simulink model "Yaw_Rate_Damper"  (R2024b)
settings: Solver=VariableStepAuto  StartTime=0.0  StopTime=40  RelTol=1e-3
undefined symbols (not defined in the file or in its folder): Kp_a
libraries: slpidlib x2
settings Model: Creator=GH-X-ST  LastModifiedBy=GH-X-ST

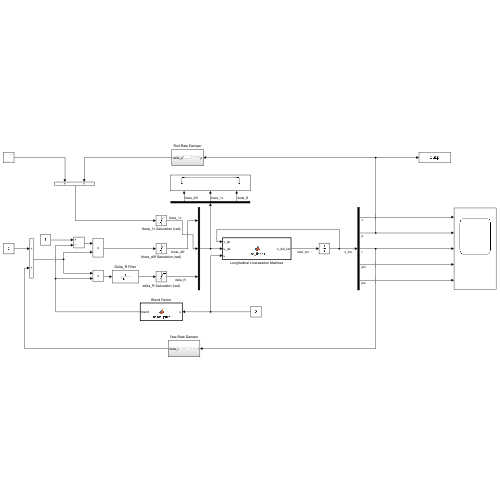
[thumbnail: Simulink's stored preview of the top-level diagram]
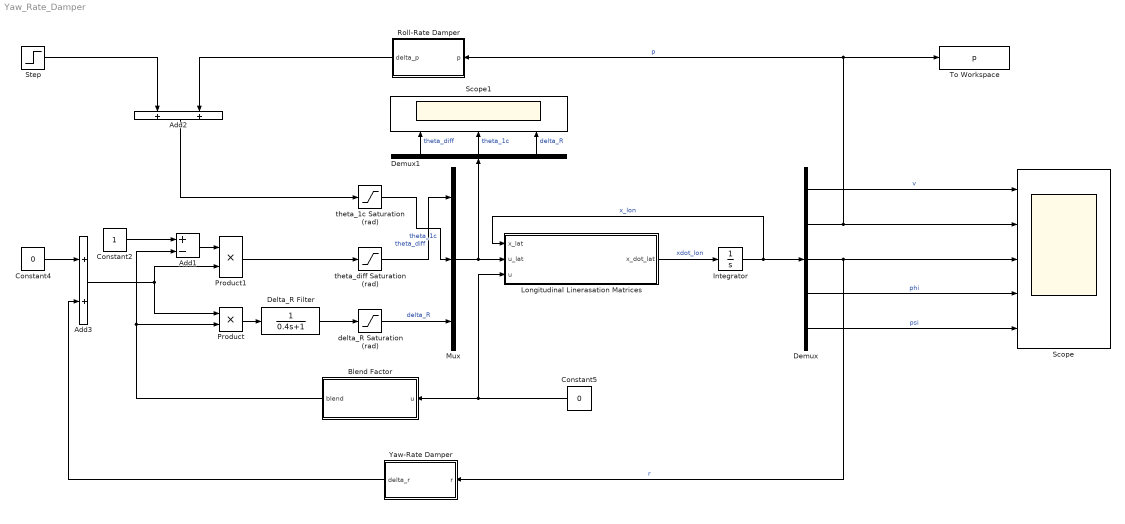
== system Yaw_Rate_Damper ==
  Add1 : Sum  Inputs=+-
  Add2 : Sum
  Add3 : Sum
  Blend Factor : MATLAB Function  TreatAsAtomicUnit=on
  Constant2 : Constant
  Constant4 : Constant  Value=0
  Constant5 : Constant  Value=0
  Delta_R Filter : TransferFcn  Denominator=[0.4 1]
  Demux : Demux  Outputs=5
  Demux1 : Demux  Outputs=3
  Integrator : Integrator  InitialCondition=[0;0;0;0;0]
  Longitudinal Linerasation Matrices : MATLAB Function  TreatAsAtomicUnit=on
  Mux : Mux  Inputs=3
  Product : Product
  Product1 : Product
  Roll-Rate Damper : Subsystem
  Scope : Scope  NumInputPorts=5
  Scope1 : Scope  NumInputPorts=3
  Step : Step  After=0.005  SampleTime=0
  To Workspace : ToWorkspace  VariableName=p  SaveFormat=Timeseries  SampleTime=-1
  Yaw-Rate Damper : Subsystem
  delta_R Saturation (rad) : Saturate  UpperLimit=deg2rad(11)  LowerLimit=deg2rad(-11)
  theta_1c Saturation (rad) : Saturate  UpperLimit=deg2rad(3)  LowerLimit=deg2rad(-3)
  theta_diff Saturation (rad) : Saturate  UpperLimit=deg2rad(5)  LowerLimit=deg2rad(-5)
  wires:
  Longitudinal Linerasation Matrices/1(x_dot_lat) -> Integrator/1  "xdot_lon"
  Integrator/1 -> Longitudinal Linerasation Matrices/1(x_lat), Demux/1  "x_lon"
  Demux/1 -> Scope/1  "v"
  Demux/2 -> Roll-Rate Damper/1(p), To Workspace/1, Scope/2  "p"
  Demux/3 -> Yaw-Rate Damper/1(r), Scope/3  "r"
  Demux/4 -> Scope/4  "phi"
  delta_R Saturation (rad)/1 -> Mux/3  "delta_R"
  Blend Factor/1(blend) -> Add1/2, Product/2
  Add3/1 -> Product1/2, Product/1
  Constant2/1 -> Add1/1
  Add1/1 -> Product1/1
  Mux/1 -> Demux1/1, Longitudinal Linerasation Matrices/2(u_lat)
  Demux1/3 -> Scope1/3  "delta_R"
  Demux1/2 -> Scope1/2  "theta_1c"
  Demux1/1 -> Scope1/1  "theta_diff"
  Product1/1 -> theta_diff Saturation (rad)/1
  Product/1 -> Delta_R Filter/1
  Delta_R Filter/1 -> delta_R Saturation (rad)/1
  Demux/5 -> Scope/5  "psi"
  Yaw-Rate Damper/1(delta_r) -> Add3/2
  Constant4/1 -> Add3/1
  theta_diff Saturation (rad)/1 -> Mux/1  "theta_diff"
  theta_1c Saturation (rad)/1 -> Mux/2  "theta_1c"
  Constant5/1 -> Longitudinal Linerasation Matrices/3(u), Blend Factor/1(u)
  Step/1 -> Add2/1
  Roll-Rate Damper/1(delta_p) -> Add2/2
  Add2/1 -> theta_1c Saturation (rad)/1

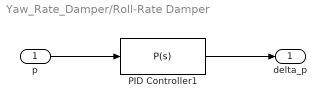
== system Yaw_Rate_Damper/Roll-Rate Damper ==
  p : Inport
  PID Controller1 : slpidlib/PID Controller  Controller=P  Form=Parallel  TimeDomain=Continuous-time  UseExternalTs=off  SampleTime=-1  IntegratorMethod=Forward Euler  FilterMethod=Forward Euler  ControllerParametersSource=internal  P=Kp_a  I=0.005  UseKiTs=off  D=0.005  UseExternalDerivativeSource=on  N=100  UseFilter=on  TunerSelectOption=Transfer Function Based (PID Tuner App)  InitialConditionSource=internal  InitialConditionForIntegrator=0  InitialConditionForFilter=0  DifferentiatorICPrevScaledInput=0  ExternalReset=none  TrackingMode=off  Kt=1  LimitOutput=on  SatLimitsSource=internal  UpperSaturationLimit=1  LowerSaturationLimit=-1  LinearizeAsGain=on  AntiWindupMode=none  Kb=1  LimitIntegrator=off  UpperIntegratorSaturationLimit=inf  LowerIntegratorSaturationLimit=-inf  POutMin=[]  POutMax=[]  IOutMin=[]  IOutMax=[]  DOutMin=[]  DOutMax=[]  NOutMin=[]  NOutMax=[]  SumOutMin=[]  SumOutMax=[]  SaturationOutMin=[]  SaturationOutMax=[]  PParamMin=[]  PParamMax=[]  IParamMin=[]  IParamMax=[]  DParamMin=[]  DParamMax=[]  NParamMin=[]  NParamMax=[]  KbParamMin=[]  KbParamMax=[]  KtParamMin=[]  KtParamMax=[]  KbOutMin=[]  KbOutMax=[]  KtOutMin=[]  KtOutMax=[]  IntegratorOutMin=[]  IntegratorOutMax=[]  FilterOutMin=[]  FilterOutMax=[]  SumI1OutMin=[]  SumI1OutMax=[]  SumI2OutMin=[]  SumI2OutMax=[]  SumI3OutMin=[]  SumI3OutMax=[]  SumI4OutMin=[]  SumI4OutMax=[]  SumDOutMin=[]  SumDOutMax=[]  DifferentiatorOutMin=[]  DifferentiatorOutMax=[]  FilterDiffOutCoefMin=[]  FilterDiffOutCoefMax=[]  ReciprocalOutMin=[]  ReciprocalOutMax=[]  SumDenOutMin=[]  SumDenOutMax=[]  SumNumOutMin=[]  SumNumOutMax=[]  DivideOutMin=[]  DivideOutMax=[]  UdiffTsProdOutMin=[]  UdiffTsProdOutMax=[]  NTsProdOutMin=[]  NTsProdOutMax=[]  UintegralTsProdOutMin=[]  UintegralTsProdOutMax=[]  UngainTsProdOutMin=[]  UngainTsProdOutMax=[]  ClampingZeroOutDataTypeStr=Inherit: Inherit via back propagation  ClampingZeroOutMin=[]  ClampingZeroOutMax=[]  FilterDenConstantOutDataTypeStr=Inherit: Inherit via back propagation  FilterDenConstantOutMin=[]  FilterDenConstantOutMax=[]  PCopyOutDataTypeStr=Inherit: Inherit via back propagation  PCopyOutMin=[]  PCopyOutMax=[]  NCopyOutDataTypeStr=Inherit: Inherit via back propagation  NCopyOutMin=[]  NCopyOutMax=[]  IntegratorContinuousStateAttributes=''  IntegratorStateMustResolveToSignalObject=off  IntegratorRTWStateStorageClass=Auto  FilterContinuousStateAttributes=''  FilterStateMustResolveToSignalObject=off  FilterRTWStateStorageClass=Auto  ParallelPVariant=InternalParameters  IdealPVariant=Disabled  IVariant=Disabled  DVariant=Disabled  IntegratorVariant=Disabled  SatVariant=Enabled  AWVariant=Disabled  PCopyVariant=Disabled  TRVariant=Disabled  FdbkBlocksVariant=Forward  IdealPFdbkVariant=Disabled  SatFdbkVariant=Disabled  DerivativeFilterVariant=Disabled  NVariant=Passthrough  NCopyVariant=Disabled_SignalSpec  FilterICVariant=Disabled  IntegratorICVariant=Disabled  ExternalResetVariant=Disabled  TRSumVariant=Passthrough  SumFdbkVariant=Disabled  SumVariant=Passthrough_P  TsampFilterVariant=InternalTs  TsampNgainVariant=Passthrough  TsampIntegralVariant=Disabled_SignalSpec  ExternalSaturationOutDataTypeStr=Inherit: Same as second input  DerivativeSourceVariant=Disabled  PreIntVariant=InternalPreInt
  delta_p : Outport
  wires:
  PID Controller1/1 -> delta_p/1
  p/1 -> PID Controller1/1

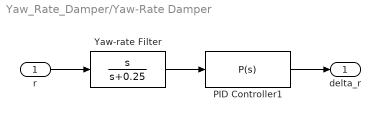
== system Yaw_Rate_Damper/Yaw-Rate Damper ==
  r : Inport
  PID Controller1 : slpidlib/PID Controller  Controller=P  Form=Parallel  TimeDomain=Continuous-time  UseExternalTs=off  SampleTime=-1  IntegratorMethod=Forward Euler  FilterMethod=Forward Euler  ControllerParametersSource=internal  P=0.01  I=0.005  UseKiTs=off  D=0.005  UseExternalDerivativeSource=on  N=100  UseFilter=on  TunerSelectOption=Transfer Function Based (PID Tuner App)  InitialConditionSource=internal  InitialConditionForIntegrator=0  InitialConditionForFilter=0  DifferentiatorICPrevScaledInput=0  ExternalReset=none  TrackingMode=off  Kt=1  LimitOutput=on  SatLimitsSource=internal  UpperSaturationLimit=1  LowerSaturationLimit=-1  LinearizeAsGain=on  AntiWindupMode=none  Kb=1  LimitIntegrator=off  UpperIntegratorSaturationLimit=inf  LowerIntegratorSaturationLimit=-inf  POutMin=[]  POutMax=[]  IOutMin=[]  IOutMax=[]  DOutMin=[]  DOutMax=[]  NOutMin=[]  NOutMax=[]  SumOutMin=[]  SumOutMax=[]  SaturationOutMin=[]  SaturationOutMax=[]  PParamMin=[]  PParamMax=[]  IParamMin=[]  IParamMax=[]  DParamMin=[]  DParamMax=[]  NParamMin=[]  NParamMax=[]  KbParamMin=[]  KbParamMax=[]  KtParamMin=[]  KtParamMax=[]  KbOutMin=[]  KbOutMax=[]  KtOutMin=[]  KtOutMax=[]  IntegratorOutMin=[]  IntegratorOutMax=[]  FilterOutMin=[]  FilterOutMax=[]  SumI1OutMin=[]  SumI1OutMax=[]  SumI2OutMin=[]  SumI2OutMax=[]  SumI3OutMin=[]  SumI3OutMax=[]  SumI4OutMin=[]  SumI4OutMax=[]  SumDOutMin=[]  SumDOutMax=[]  DifferentiatorOutMin=[]  DifferentiatorOutMax=[]  FilterDiffOutCoefMin=[]  FilterDiffOutCoefMax=[]  ReciprocalOutMin=[]  ReciprocalOutMax=[]  SumDenOutMin=[]  SumDenOutMax=[]  SumNumOutMin=[]  SumNumOutMax=[]  DivideOutMin=[]  DivideOutMax=[]  UdiffTsProdOutMin=[]  UdiffTsProdOutMax=[]  NTsProdOutMin=[]  NTsProdOutMax=[]  UintegralTsProdOutMin=[]  UintegralTsProdOutMax=[]  UngainTsProdOutMin=[]  UngainTsProdOutMax=[]  ClampingZeroOutDataTypeStr=Inherit: Inherit via back propagation  ClampingZeroOutMin=[]  ClampingZeroOutMax=[]  FilterDenConstantOutDataTypeStr=Inherit: Inherit via back propagation  FilterDenConstantOutMin=[]  FilterDenConstantOutMax=[]  PCopyOutDataTypeStr=Inherit: Inherit via back propagation  PCopyOutMin=[]  PCopyOutMax=[]  NCopyOutDataTypeStr=Inherit: Inherit via back propagation  NCopyOutMin=[]  NCopyOutMax=[]  IntegratorContinuousStateAttributes=''  IntegratorStateMustResolveToSignalObject=off  IntegratorRTWStateStorageClass=Auto  FilterContinuousStateAttributes=''  FilterStateMustResolveToSignalObject=off  FilterRTWStateStorageClass=Auto  ParallelPVariant=InternalParameters  IdealPVariant=Disabled  IVariant=Disabled  DVariant=Disabled  IntegratorVariant=Disabled  SatVariant=Enabled  AWVariant=Disabled  PCopyVariant=Disabled  TRVariant=Disabled  FdbkBlocksVariant=Forward  IdealPFdbkVariant=Disabled  SatFdbkVariant=Disabled  DerivativeFilterVariant=Disabled  NVariant=Passthrough  NCopyVariant=Disabled_SignalSpec  FilterICVariant=Disabled  IntegratorICVariant=Disabled  ExternalResetVariant=Disabled  TRSumVariant=Passthrough  SumFdbkVariant=Disabled  SumVariant=Passthrough_P  TsampFilterVariant=InternalTs  TsampNgainVariant=Passthrough  TsampIntegralVariant=Disabled_SignalSpec  ExternalSaturationOutDataTypeStr=Inherit: Same as second input  DerivativeSourceVariant=Disabled  PreIntVariant=InternalPreInt
  Yaw-rate Filter : TransferFcn  Numerator=[1 0]  Denominator=[1 0.25]
  delta_r : Outport
  wires:
  PID Controller1/1 -> delta_r/1
  Yaw-rate Filter/1 -> PID Controller1/1
  r/1 -> Yaw-rate Filter/1

== matlab function Yaw_Rate_Damper/Longitudinal Linerasation Matrices ==
  data: x_lat input; u_lat input; u input; x_dot_lat output
function x_dot_lat = Lat_linear(x_lat, u_lat, u)
% Author:
%   Hanchen Li (hl3422@ic.ac.uk)
%
% Inputs:
%   x_lat     - [v, p, r, phi, psi]
%   v         - Lateral velocity (m/s)
%   p         - Roll rate (rad/s)
%   r         - Yaw rate (rad/s)
%   phi       - Euler roll angle (rad)
%   psi       - Euler yaw angle (rad)
%
%   u_lat      - [theta_diff, theta_1c, delta_R]
%   theta_diff - Rotor collective difference (rad)
%   theta_1c   - Lateral cyclic (rad)
%   delta_R    - Rudder deflection (rad)
%
%   u         - Forward velocity (m/s)
%
% Outputs:
%   x_dot_lat

A_lat = ...
[-0.00723803596901745	0.766629187912504	0	9.80664998365558	0;
        -0.0220588605968897	2.33772683898305	0	0	0;
        -0.00849763594524569	0.895100650677353	0	0	0;
        0	1	-3.37129866355175e-20	0	0;
        0	0	1	0	0];

B_lat = ...
[3.23169927067643e-19	-5.17979000748556	0;
        39.4348460540525	-15.7950340421649	0;
        20.0367522163849	-6.04781748357008	0;
        0	0	0;
        0	0	0];

%% 3 Output
x_dot_lat = A_lat * x_lat + B_lat * u_lat;

end

== matlab function Yaw_Rate_Damper/Blend Factor ==
  data: blend output; u input
function blend = Blend_pitch(u)
% Author:
%   Hanchen Li (hl3422@ic.ac.uk)
%
% Inputs:
%   u         - Forward velocity (m/s)
%
% Outputs:
%   blend     - blend factor

%% 1 Decide blend factor

if abs(u) < 1e-4

    blend = 0;

elseif abs(u) < 90.3

    blend = u / (90.3 / 0.8);

else

    blend = 0.8;

end

end
